simulink model "untitled"  (R2024a)
settings: Solver=VariableStepAuto  StartTime=0.0  StopTime=10.0  RelTol=1e-3
settings Model: PacingRate=1.100000  Creator=Asus  LastModifiedBy=Asus

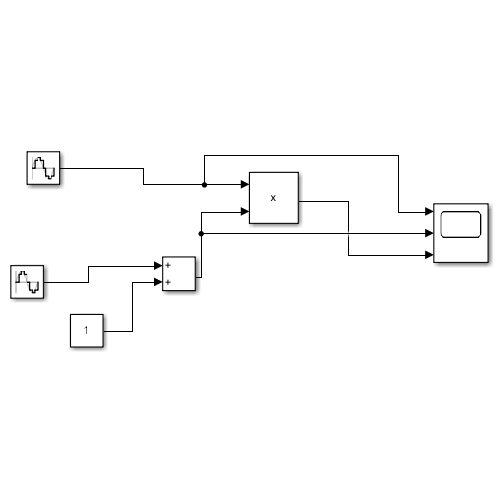
[thumbnail: Simulink's stored preview of the top-level diagram]
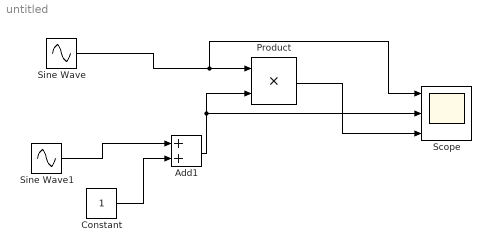
== system untitled ==
  Add1 : Sum
  Constant : Constant
  Product : Product
  Scope : Scope  NumInputPorts=3
  Sine Wave : Sin  Amplitude=2  Frequency=20  SampleTime=0.001
  Sine Wave1 : Sin  Frequency=2  SampleTime=0.001
  wires:
  Constant/1 -> Add1/2
  Sine Wave1/1 -> Add1/1
  Add1/1 -> Scope/2, Product/2
  Sine Wave/1 -> Scope/1, Product/1
  Product/1 -> Scope/3
